simulink model "Linearized_model"  (R2019b)
settings: Solver=VariableStepAuto  StartTime=0.0  StopTime=15  RelTol=1e-6
undefined symbols (not defined in the file or in its folder): D_e, dD0, dE0, dI0, dJ0, dR0, dS0, R_e, S_e, u_e
settings Model: Creator=felipeareces  LastModifiedBy=felipeareces

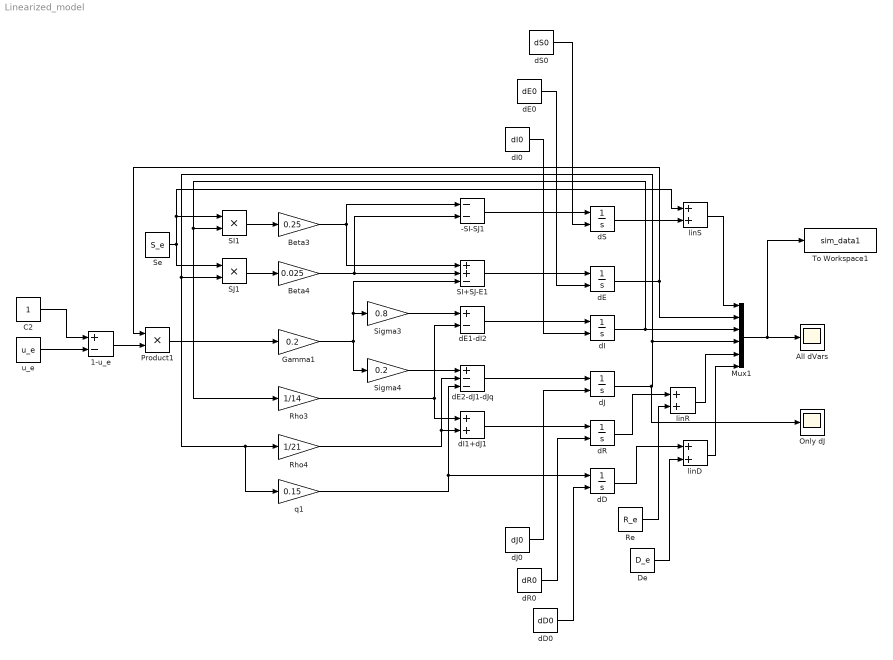
== system Linearized_model ==
  -SI-SJ1 : Sum  Inputs=--
  1-u_e : Sum  Inputs=+-
  All dVars : Scope
  Beta3 : Gain  Gain=0.25
  Beta4 : Gain  Gain=0.025
  C2 : Constant
  De : Constant  Value=D_e
  Gamma1 : Gain  Gain=0.2
  Mux1 : Mux  Inputs=6
  Only dJ : Scope
  Product1 : Product
  Re : Constant  Value=R_e
  Rho3 : Gain  Gain=1/14
  Rho4 : Gain  Gain=1/21
  SI+SJ-E1 : Sum  Inputs=++-
  SI1 : Product
  SJ1 : Product
  Se : Constant  Value=S_e
  Sigma3 : Gain  Gain=0.8
  Sigma4 : Gain  Gain=0.2
  To Workspace1 : ToWorkspace  VariableName=sim_data1  SaveFormat=Timeseries  SampleTime=-1
  dD : Integrator  InitialConditionSource=external
  dD0 : Constant  Value=dD0
  dE : Integrator  InitialConditionSource=external
  dE0 : Constant  Value=dE0
  dE1-dI2 : Sum  Inputs=+-
  dE2-dJ1-dJq : Sum  Inputs=+--
  dI : Integrator  InitialConditionSource=external
  dI0 : Constant  Value=dI0
  dI1+dJ1 : Sum
  dJ : Integrator  InitialConditionSource=external
  dJ0 : Constant  Value=dJ0
  dR : Integrator  InitialConditionSource=external
  dR0 : Constant  Value=dR0
  dS : Integrator  InitialConditionSource=external
  dS0 : Constant  Value=dS0
  linD : Sum
  linR : Sum
  linS : Sum
  q1 : Gain  Gain=0.15
  u_e : Constant  Value=u_e
  wires:
  u_e/1 -> 1-u_e/2
  dE1-dI2/1 -> dI/1
  q1/1 -> dE2-dJ1-dJq/3, dD/1
  Beta3/1 -> SI+SJ-E1/1, -SI-SJ1/1
  C2/1 -> 1-u_e/1
  dE2-dJ1-dJq/1 -> dJ/1
  1-u_e/1 -> Product1/2
  dE/1 -> Product1/1, Mux1/2
  Mux1/1 -> To Workspace1/1, All dVars/1
  SI+SJ-E1/1 -> dE/1
  dD0/1 -> dD/2
  Product1/1 -> Gamma1/1
  dR0/1 -> dR/2
  SJ1/1 -> Beta4/1
  dJ0/1 -> dJ/2
  Sigma3/1 -> dE1-dI2/1
  Rho4/1 -> dE2-dJ1-dJq/2, dI1+dJ1/2
  -SI-SJ1/1 -> dS/1
  Rho3/1 -> dE1-dI2/2, dI1+dJ1/1
  Sigma4/1 -> dE2-dJ1-dJq/1
  dI1+dJ1/1 -> dR/1
  dI0/1 -> dI/2
  dS0/1 -> dS/2
  dE0/1 -> dE/2
  Beta4/1 -> -SI-SJ1/2, SI+SJ-E1/2
  SI1/1 -> Beta3/1
  dI/1 -> Mux1/3, Rho3/1, SI1/2
  dJ/1 -> Only dJ/1, Mux1/4, q1/1, Rho4/1, SJ1/2
  Gamma1/1 -> Sigma4/1, SI+SJ-E1/3, Sigma3/1
  Se/1 -> linS/1, SI1/1, SJ1/1
  dS/1 -> linS/2
  linS/1 -> Mux1/1
  De/1 -> linD/2
  Re/1 -> linR/2
  dR/1 -> linR/1
  dD/1 -> linD/1
  linR/1 -> Mux1/5
  linD/1 -> Mux1/6
